simulink model "ssc_solenoid"  (R2022a)
settings: Solver=VariableStepAuto  StartTime=0.0  StopTime=2  MaxStep=0.01  RelTol=1e-3  AbsTol=1e-3  EnableMultiTasking=on
libraries: fl_lib x26, nesl_utility x4
CloseFcn:
  | try,close(h1_ssc_solenoid),end
  | clear h1_ssc_solenoid
  | 
  | clear simlog_ssc_solenoid
Description:
  | Solenoid
settings Model: Creator=The MathWorks, Inc.  LastModifiedBy=whatastarrynight
settings SolverCC: AutoScaleAbsTol=off  AlgebraicLoopSolver=TrustRegion
settings DataIOCC: LimitDataPoints=on  SaveFormat=Array  ReturnWorkspaceOutputs=off
settings OptimizationCC: LifeSpan=inf
settings DebuggingCC: SolverPrmCheckMsg=warning  UnconnectedInputMsg=warning  UnconnectedOutputMsg=warning  UnconnectedLineMsg=warning  AllowSymbolicDim=off  PregeneratedLibrarySubsystemCodeDiagnostic=none  SFUnexpectedBacktrackingDiag=warning  SFNoUnconditionalDefaultTransitionDiag=warning  SFExecutionAtInitializationDiag=none  SFMachineParentedDataDiag=warning  ArithmeticOperatorsInVariantConditions=warning
settings HardwareCC: ProdBitPerPointer=32  ProdBitPerSizeT=32  ProdBitPerPtrDiffT=32  ProdLargestAtomicFloat=None  ProdIntDivRoundTo=Undefined  ProdEndianess=Unspecified  ProdWordSize=32  ProdHWDeviceType=32-bit Generic
settings ModelReferenceCC: PropagateSignalLabelsOutOfModel=off
settings SFSimCC: SimUseLocalCustomCode=off  CustomCodeUndefinedFunction=UseInterfaceOnly
settings RTWCC: RTWUseLocalCustomCode=off  DLArmComputeVersion=19.05
settings CodeAppCC: StateflowObjectComments=on
settings GRTTargetCC: TargetLangStandard=C89/C90 (ANSI)
settings ConfigComp: CovMetricSettings=dw  CovSaveCumulativeToWorkspaceVar=on  CovSaveSingleToWorkspaceVar=on  CovExternalEMLEnable=off  CovSFcnEnable=off
settings SimscapeCC: SimscapeLogType=all  SimscapeLogSimulationStatistics=on  SimscapeLogName=simlog_ssc_solenoid  SimscapeLogDataHistory=10000

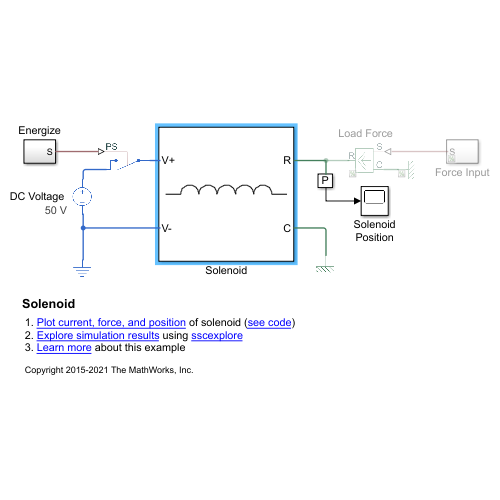
[thumbnail: Simulink's stored preview of the top-level diagram]
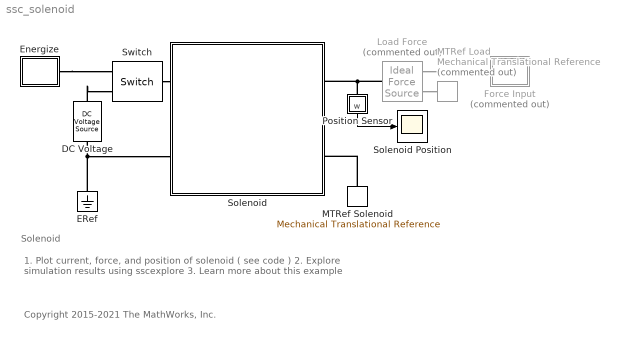
== system ssc_solenoid ==
  note: 1. Plot current, force, and position of solenoid ( see code )
      | 2. Explore simulation results using sscexplore
      | 3. Learn more about this example
  note: Solenoid
  note: Copyright 2015-2021 The MathWorks, Inc.
  DC Voltage : fl_lib/Electrical/Electrical Sources/DC Voltage Source  v0=50 V
      settings: AttributesFormatString=%<v0> %<v0_unit>  SourceProductBaseCode=PW,SS,VE
  ERef : fl_lib/Electrical/Electrical Elements/Electrical Reference
      settings: SourceProductBaseCode=PW,SS,VE
  Energize : Subsystem
  Force Input : Subsystem  Commented=on
  Load Force : fl_lib/Mechanical/Mechanical Sources/Ideal Force Source  Commented=on
      settings: SourceProductBaseCode=PW,SS,VE
  MTRef Load : fl_lib/Mechanical/Translational Elements/Mechanical Translational Reference  Commented=on
      settings: SourceProductBaseCode=PW,SS,VE
  MTRef Solenoid : fl_lib/Mechanical/Translational Elements/Mechanical Translational Reference
      settings: SourceProductBaseCode=PW,SS,VE
  Position Sensor : Subsystem
      mask Display: disp('P');
  Solenoid : Subsystem  Tag=PublishSubsystem
      mask Display:
      | plot(sin(-pi/2:0.1:pi/2)*0.15+0.6,cos(-pi/2:0.1:pi/2)*0.15+0);
      | plot(sin(-pi/2:0.1:pi/2)*0.15+0.3,cos(-pi/2:0.1:pi/2)*0.15+0);
      | plot(sin(-pi/2:0.1:pi/2)*0.15+0.0,cos(-pi/2:0.1:pi/2)*0.15+0);
      | plot(sin(-pi/2:0.1:pi/2)*0.15-0.3,cos(-pi/2:0.1:pi/2)*0.15+0);
      | plot(sin(-pi/2:0.1:pi/2)*0.15-0.6,cos(-pi/2:0.1:pi/2)*0.15+0);
      | plot([-1.0 -0.75],[0 0]);
      | plot([1.0 0.75],[0 0]);
      | 
      | % Plot points to set plot range
      | color('white');plot(1.1,1.1);plot(-1.1,-1.1)
      | color('black');
      | 
      | port_label('RConn',1,'R');
      | port_label('RConn',2,'C');
      | port_label('LConn',1,'V+');
      | port_label('LConn',2,'V-');
  Solenoid Position : Scope
  Switch : fl_lib/Electrical/Electrical Elements/Switch  R_closed=0.01 Ohm  G_open=1e-08 1/Ohm  Threshold=0  i_specify=off  i_priority=High  i=0 A  i_nominal_specify=off  i_nominal_unit=A  i_nominal_value=1  v_specify=off  v_priority=High  v=0 V  v_nominal_specify=off  v_nominal_unit=V  v_nominal_value=1
      settings: SourceProductBaseCode=PW,SS,VE
  wires:
  Position Sensor/1(w) -> Solenoid Position/1
  connections:
  ERef/LConn1 -- Solenoid/LConn2 -- DC Voltage/RConn1
  Switch/LConn1 -- Solenoid/LConn1
  DC Voltage/LConn1 -- Switch/RConn2
  Load Force/RConn2 -- MTRef Load/LConn1
  Position Sensor/LConn1 -- Solenoid/RConn1 -- Load Force/LConn1
  MTRef Solenoid/LConn1 -- Solenoid/RConn2
  Energize/RConn1 -- Switch/RConn1
  Load Force/RConn1 -- Force Input/LConn1

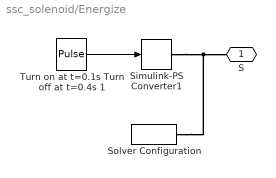
== system ssc_solenoid/Energize ==
  Simulink-PS Converter1 : nesl_utility/Simulink-PS Converter  PhysicalDomain=network_engine_domain  SubClassName=ps_input  LeftPortType=input  RightPortType=output  PseudoPeriodic=off  Frequencies=[]  NoiseDistribution=none  NoiseParameters=[]  Unit=1  AffineConversion=off  FilteringAndDerivatives=zero  SimscapeFilterOrder=1  InputFilterTimeConstant=.001  UdotUserProvided=[]
      settings: SourceProductBaseCode=SS,PW,VE
  Solver Configuration : nesl_utility/Solver Configuration  PhysicalDomain=network_engine_domain  SubClassName=solver  LeftPortType=input  RightPortType=generic  Tones=[]  Harmonics=[]  SimulateNoise=off  Profile=off  UseLocalSampling=off  EnableSwitchedLinearOptims=on  FrequencyDomain=off  UseCCode=off  RelTol=0.001  AbsTol=1e-06  MinStep=1e-09  ToWorkspace=off  RevertToSquareIcSolve=off  NumHomotopyIterations=100  PhasorMode=off  PhasorModeNumHarmonics=1  IndexReductionMethod=DerivativeReplacement  DoDC=off  ResidualTolerance=1e-9  UseLocalSolver=off  LocalSolverChoice=NE_BACKWARD_EULER_ADVANCER  LocalSolverSampleTime=.001  DoFixedCost=off  MaxNonlinIter=3  MaxModeIter=2  ComputeImpulses=off  ImpulseIterations=2  LinearAlgebra=auto  LinearAlgebraNumThread=0  EquationFormulation=NE_TIME_EF  DelaysMemoryBudget=1024  AutomaticFiltering=on  FilteringTimeConstant=0.001  PartitionStorageMethod=AS_NEEDED  PartitionMemoryBudget=1024  PartitionMethod=FAST
      settings: SourceProductBaseCode=SS,PW,VE
  Turn on at t=0.1s Turn off at t=0.4s 1 : DiscretePulseGenerator  PulseType=Time based  PulseWidth=15  PhaseDelay=0.1
  S : PMIOPort  Side=Right
  wires:
  Turn on at t=0.1s Turn off at t=0.4s 1/1 -> Simulink-PS Converter1/1
  connections:
  Simulink-PS Converter1/RConn1 -- Solver Configuration/RConn1 -- S/RConn1

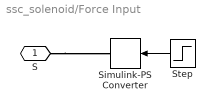
== system ssc_solenoid/Force Input ==
  Simulink-PS Converter : nesl_utility/Simulink-PS Converter  PhysicalDomain=network_engine_domain  SubClassName=ps_input  LeftPortType=input  RightPortType=output  PseudoPeriodic=off  Frequencies=[]  NoiseDistribution=none  NoiseParameters=[]  Unit=1  AffineConversion=off  FilteringAndDerivatives=zero  SimscapeFilterOrder=1  InputFilterTimeConstant=.001  UdotUserProvided=[]
      settings: SourceProductBaseCode=SS,PW,VE
  Step : Step  Time=0.3  After=10  SampleTime=0
  S : PMIOPort  Side=Left
  wires:
  Step/1 -> Simulink-PS Converter/1
  connections:
  S/RConn1 -- Simulink-PS Converter/RConn1

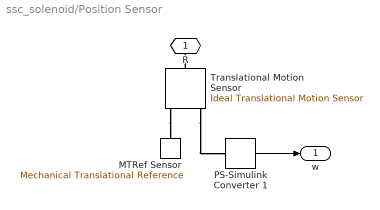
== system ssc_solenoid/Position Sensor ==
  MTRef Sensor : fl_lib/Mechanical/Translational Elements/Mechanical Translational Reference
      settings: SourceProductBaseCode=PW,SS,VE
  PS-Simulink Converter 1 : nesl_utility/PS-Simulink Converter  PhysicalDomain=network_engine_domain  SubClassName=ps_output  LeftPortType=input  RightPortType=output  PseudoPeriodic=off  Frequencies=[]  VectorFormat=1-D array  Unit=mm  AffineConversion=off
      settings: SourceProductBaseCode=SS,PW,VE
  Translational Motion Sensor : fl_lib/Mechanical/Mechanical Sensors/Ideal Translational Motion Sensor  offset=5 mm
      settings: SourceProductBaseCode=PW,SS,VE
  R : PMIOPort  Side=Left
  w : Outport  VectorParamsAs1DForOutWhenUnconnected=off
  wires:
  PS-Simulink Converter 1/1 -> w/1
  connections:
  Translational Motion Sensor/RConn3 -- PS-Simulink Converter 1/LConn1
  Translational Motion Sensor/RConn1 -- MTRef Sensor/LConn1
  Translational Motion Sensor/LConn1 -- R/RConn1

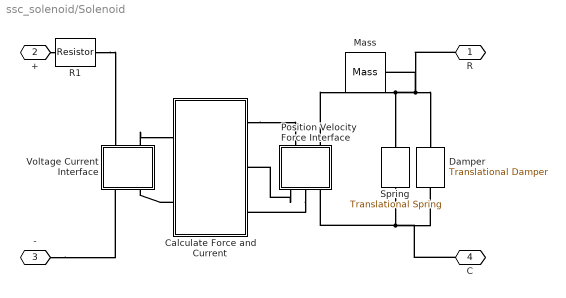
== system ssc_solenoid/Solenoid ==
  Calculate Force and Current : Subsystem
  Damper : fl_lib/Mechanical/Translational Elements/Translational Damper  D=20 N/(m/s)  v_specify=off  v_priority=High  v=0 m/s  v_nominal_specify=off  v_nominal_unit=m/s  v_nominal_value=1  f_specify=off  f_priority=High  f=0 N  f_nominal_specify=off  f_nominal_unit=N  f_nominal_value=1
      settings: SourceProductBaseCode=PW,SS,VE
  Mass : fl_lib/Mechanical/Translational Elements/Mass  mass=0.1 kg  num_ports=foundation.enum.numPorts2.one  v_specify=off  v_priority=High  v=0 m/s  v_nominal_specify=off  v_nominal_unit=m/s  v_nominal_value=1  f_specify=off  f_priority=High  f=0 N  f_nominal_specify=off  f_nominal_unit=N  f_nominal_value=1
      settings: SourceProductBaseCode=PW,SS,VE
  Position Velocity Force Interface : Subsystem
  R1 : fl_lib/Electrical/Electrical Elements/Resistor  R=1000 Ohm  i_specify=off  i_priority=High  i=0 A  i_nominal_specify=off  i_nominal_unit=A  i_nominal_value=1  v_specify=off  v_priority=High  v=0 V  v_nominal_specify=off  v_nominal_unit=V  v_nominal_value=1
      settings: SourceProductBaseCode=PW,SS,VE
  Spring : fl_lib/Mechanical/Translational Elements/Translational Spring  spr_rate=200 N/m  v_specify=off  v_priority=High  v=0 m/s  v_nominal_specify=off  v_nominal_unit=m/s  v_nominal_value=1  f_specify=off  f_priority=High  f=0 N  f_nominal_specify=off  f_nominal_unit=N  f_nominal_value=1  x_specify=off  x_priority=High  x=0 mm  x_nominal_specify=off  x_nominal_unit=m  x_nominal_value=1
      settings: SourceProductBaseCode=PW,SS,VE
  Voltage Current Interface : Subsystem
  R : PMIOPort  Side=Right
  + : PMIOPort  Port=2  Side=Left
  - : PMIOPort  Port=3  Side=Left
  C : PMIOPort  Port=4  Side=Right
  connections:
  R/RConn1 -- Mass/LConn1 -- Damper/LConn1 -- Position Velocity Force Interface/LConn2 -- Spring/LConn1
  Spring/RConn1 -- Damper/RConn1 -- C/RConn1 -- Position Velocity Force Interface/RConn3
  +/RConn1 -- R1/LConn1
  Calculate Force and Current/RConn1 -- Position Velocity Force Interface/LConn1
  Position Velocity Force Interface/RConn1 -- Calculate Force and Current/RConn2
  Position Velocity Force Interface/RConn2 -- Calculate Force and Current/RConn3
  R1/RConn1 -- Voltage Current Interface/LConn1
  Calculate Force and Current/LConn2 -- Voltage Current Interface/RConn2
  Voltage Current Interface/LConn2 -- Calculate Force and Current/LConn1
  -/RConn1 -- Voltage Current Interface/RConn1

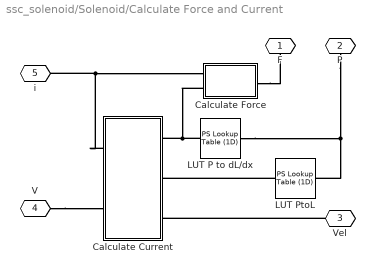
== system ssc_solenoid/Solenoid/Calculate Force and Current ==
  Calculate Current : Subsystem
  Calculate Force : Subsystem
  LUT P to dL/dx : fl_lib/Physical Signals/Lookup Tables/PS Lookup Table (1D)  x="[-0.0200   -0.0100   -0.0050   -0.0020   -0.0010     -0.0001    0   0.0001    0.0010    0.0020    0.0050    0.0100    0.0200] m"  f="1e3*[0.0339    0.1282    0.4592    2.1302    5.6250  25.6250       0  -25.6250 -5.6250   -2.1302   -0.4592   -0.1282   -0.0339] H/m"  interp_method=simscape.enum.interpolation.linear  extrap_method=simscape.enum.extrapolation.linear
      settings: SourceProductBaseCode=PW,SS,VE
  LUT PtoL : fl_lib/Physical Signals/Lookup Tables/PS Lookup Table (1D)  x="[-0.0200   -0.0100   -0.0050   -0.0020   -0.0010         0    0.0010    0.0020    0.0050    0.0100    0.0200] m"  f="[0.6990    1.3585    2.5714    5.5385    9.0000   24.0000    9.0000    5.5385    2.5714    1.3585    0.6990] H"  interp_method=simscape.enum.interpolation.linear  extrap_method=simscape.enum.extrapolation.linear
      settings: SourceProductBaseCode=PW,SS,VE
  F : PMIOPort  Side=Right
  P : PMIOPort  Port=2  Side=Right
  Vel : PMIOPort  Port=3  Side=Right
  V : PMIOPort  Port=4  Side=Left
  i : PMIOPort  Port=5  Side=Left
  connections:
  Calculate Force/RConn1 -- F/RConn1
  Calculate Force/LConn2 -- LUT P to dL/dx/RConn1 -- Calculate Current/LConn1
  V/RConn1 -- Calculate Current/RConn2
  Vel/RConn1 -- Calculate Current/LConn3
  Calculate Current/RConn1 -- i/RConn1 -- Calculate Force/LConn1
  LUT P to dL/dx/LConn1 -- LUT PtoL/LConn1 -- P/RConn1
  LUT PtoL/RConn1 -- Calculate Current/LConn2

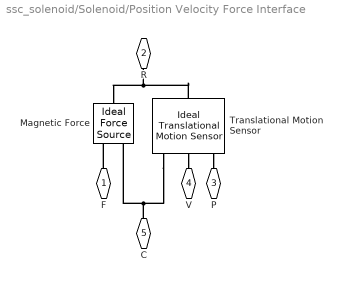
== system ssc_solenoid/Solenoid/Position Velocity Force Interface ==
  Magnetic Force : fl_lib/Mechanical/Mechanical Sources/Ideal Force Source
      settings: SourceProductBaseCode=PW,SS,VE
  Translational Motion Sensor : fl_lib/Mechanical/Mechanical Sensors/Ideal Translational Motion Sensor  offset=5 mm
      settings: SourceProductBaseCode=PW,SS,VE
  F : PMIOPort  Side=Left
  R : PMIOPort  Port=2  Side=Left
  P : PMIOPort  Port=3  Side=Right
  V : PMIOPort  Port=4  Side=Right
  C : PMIOPort  Port=5  Side=Right
  connections:
  Translational Motion Sensor/RConn1 -- C/RConn1 -- Magnetic Force/RConn2
  Translational Motion Sensor/LConn1 -- R/RConn1 -- Magnetic Force/LConn1
  Translational Motion Sensor/RConn2 -- V/RConn1
  Translational Motion Sensor/RConn3 -- P/RConn1
  F/RConn1 -- Magnetic Force/RConn1

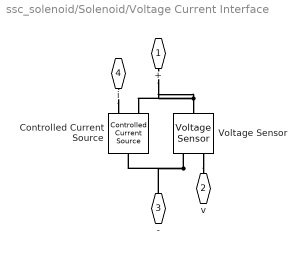
== system ssc_solenoid/Solenoid/Voltage Current Interface ==
  Controlled Current Source : fl_lib/Electrical/Electrical Sources/Controlled Current Source
      settings: SourceProductBaseCode=PW,SS,VE
  Voltage Sensor : fl_lib/Electrical/Electrical Sensors/Voltage Sensor
      settings: SourceProductBaseCode=PW,SS,VE
  + : PMIOPort  Side=Left
  v : PMIOPort  Port=2  Side=Left
  - : PMIOPort  Port=3  Side=Right
  i : PMIOPort  Port=4  Side=Right
  connections:
  Voltage Sensor/RConn1 -- v/RConn1
  i/RConn1 -- Controlled Current Source/RConn1
  Voltage Sensor/LConn1 -- Controlled Current Source/RConn2 -- +/RConn1
  Voltage Sensor/RConn2 -- Controlled Current Source/LConn1 -- -/RConn1

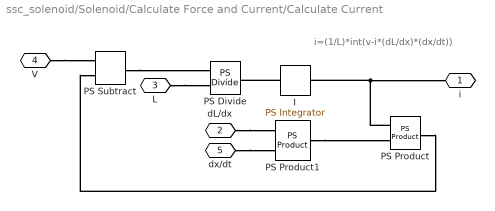
== system ssc_solenoid/Solenoid/Calculate Force and Current/Calculate Current ==
  note: i=(1/L)*int(v-i*(dL/dx)*(dx/dt))
  I : fl_lib/Physical Signals/Linear Operators/PS Integrator  reset_method=foundation.enum.IntegratorResetSpec.None  initial_condition_spec=foundation.enum.IntegratorICSpec.Internal  x0=0 A
      settings: SourceProductBaseCode=PW,SS,VE
  PS Divide : fl_lib/Physical Signals/Functions/PS Divide
      settings: SourceProductBaseCode=PW,SS,VE
  PS Product : fl_lib/Physical Signals/Functions/PS Product
      settings: SourceProductBaseCode=PW,SS,VE
  PS Product1 : fl_lib/Physical Signals/Functions/PS Product
      settings: SourceProductBaseCode=PW,SS,VE
  PS Subtract : fl_lib/Physical Signals/Functions/PS Subtract
      settings: SourceProductBaseCode=PW,SS,VE
  i : PMIOPort  Side=Right
  dL/dx : PMIOPort  Port=2  Side=Left
  L : PMIOPort  Port=3  Side=Left
  V : PMIOPort  Port=4  Side=Right
  dx/dt : PMIOPort  Port=5  Side=Left
  connections:
  I/LConn1 -- PS Divide/RConn1
  PS Subtract/RConn1 -- PS Divide/LConn1
  PS Product1/RConn1 -- PS Product/LConn2
  PS Product/RConn1 -- PS Subtract/LConn2
  L/RConn1 -- PS Divide/LConn2
  V/RConn1 -- PS Subtract/LConn1
  dL/dx/RConn1 -- PS Product1/LConn1
  dx/dt/RConn1 -- PS Product1/LConn2
  PS Product/LConn1 -- i/RConn1 -- I/RConn1

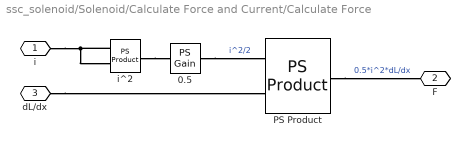
== system ssc_solenoid/Solenoid/Calculate Force and Current/Calculate Force ==
  0.5 : fl_lib/Physical Signals/Functions/PS Gain  gain=0.5
      settings: SourceProductBaseCode=PW,SS,VE
  PS Product : fl_lib/Physical Signals/Functions/PS Product
      settings: SourceProductBaseCode=PW,SS,VE
  i^2 : fl_lib/Physical Signals/Functions/PS Product
      settings: SourceProductBaseCode=PW,SS,VE
  i : PMIOPort  Side=Left
  F : PMIOPort  Port=2  Side=Right
  dL/dx : PMIOPort  Port=3  Side=Left
  connections:
  i^2/LConn1 -- i^2/LConn2 -- i/RConn1
  PS Product/RConn1 -- F/RConn1  "0.5*i^2*dL/dx"
  dL/dx/RConn1 -- PS Product/LConn2
  i^2/RConn1 -- 0.5/LConn1
  0.5/RConn1 -- PS Product/LConn1  "i^2/2"
